simulink model "mdl_GPSreceiveBin1_monitor_v2"  (R2020b)
settings: Solver=FixedStepDiscrete  StartTime=0.0  StopTime=5  FixedStep=0.01  RelTol=1e-3  EnableMultiTasking=on
libraries: simulink x4, raspberrypiCommlib x1
settings Model: ModifiedByFormat=The MathWorks Inc.  SimulationMode=external  EnablePacing=on  Creator=The MathWorks, Inc.  LastModifiedBy=The MathWorks Inc.
settings SolverCC: PositivePriorityOrder=on
settings DataIOCC: SaveFormat=Array  SaveOutput=off  DSMLogging=off  ReturnWorkspaceOutputs=off
settings OptimizationCC: LifeSpan=1  MaxStackSize=64
settings DebuggingCC: UnderspecifiedInitializationDetection=Classic  MergeDetectMultiDrivingBlocksExec=none  SolverPrmCheckMsg=warning  AllowSymbolicDim=off  SFUnexpectedBacktrackingDiag=warning  SFNoUnconditionalDefaultTransitionDiag=warning  SFExecutionAtInitializationDiag=none  ArithmeticOperatorsInVariantConditions=warning
settings HardwareCC: ProdBitPerPointer=32  ProdBitPerSizeT=32  ProdBitPerPtrDiffT=32  ProdLargestAtomicInteger=Long  ProdLargestAtomicFloat=Double  ProdWordSize=32  ProdHWDeviceType=ARM Compatible->ARM Cortex
settings ModelReferenceCC: PropagateSignalLabelsOutOfModel=off
settings SFSimCC: SimUseLocalCustomCode=off  MATLABDynamicMemAlloc=off  CustomCodeUndefinedFunction=UseInterfaceOnly
settings RTWCC: Description=Embedded Coder  SystemTargetFile=ert.tlc  HardwareBoard=Raspberry Pi  TemplateMakefile=ert_default_tmf  RTWVerbose=off  RTWUseLocalCustomCode=off  Toolchain=GNU GCC Raspberry Pi
settings CodeAppCC: MangleLength=10  StateflowObjectComments=on
settings ERTTargetCC: MultiwordLength=2048  ERTCustomFileBanners=off  MatFileLogging=on  SupportContinuousTime=on  RemoveResetFunc=off  SupportVariableSizeSignals=on  ModelStepFunctionPrototypeControlCompliant=off  ExtMode=on  ExtModeTransport=2  ExtModeStaticAlloc=on  ExtModeMexFile=ext_xcp  ExtModeMexArgs='FlexCase04.local' 1 17725  ExtModeIntrfLevel=Level2 - Open  ERTSrcFileBannerTemplate=codertarget_code_template.cgt  ERTHdrFileBannerTemplate=codertarget_code_template.cgt  ERTDataSrcFileTemplate=codertarget_code_template.cgt  ERTDataHdrFileTemplate=codertarget_code_template.cgt  ConvertIfToSwitch=off  SuppressUnreachableDefaultCases=off
settings ConfigComp: CovMetricSettings=dw  CovSaveCumulativeToWorkspaceVar=on  CovSaveSingleToWorkspaceVar=on  CovExternalEMLEnable=off  CovSFcnEnable=off

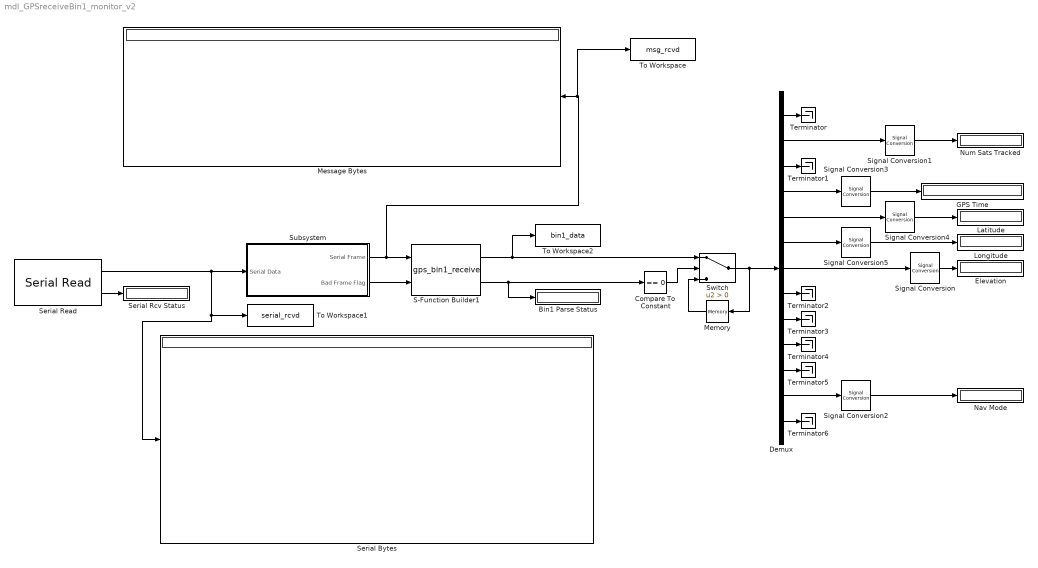
== system mdl_GPSreceiveBin1_monitor_v2 ==
  Bin1 Parse Status : Display
  Compare To Constant : simulink/Logic and Bit Operations/Compare To Constant  relop===  const=0  OutDataTypeStr=uint8
  Demux : Demux  Outputs=13
  Elevation : Display
  GPS Time : Display
      settings: Format=long_e
  Latitude : Display
  Longitude : Display
  Memory : Memory  InheritSampleTime=on  LinearizeAsDelay=on
  Message Bytes : Display
      settings: Format=hex (Stored Integer)
  Nav Mode : Display
  Num Sats Tracked : Display
  S-Function Builder1 : S-Function  FunctionName=gps_bin1_receive  SFunctionModules=gps_bin1_receive_wrapper  SFunctionDeploymentMode=off  EnableBusSupport=off  mask(S-Function Builder){}
      mask help: Simulink:masks:SFunctionBuilder_MD
      mask init:
      | val = [[.9  0.75 0.75 1 1 .9 .9 1]',[1 1 0.75 0.75 .9 .9 1 .9]'];try , sys = get_param(gcb,'SfunBuilderFcnName');if isempty(sys), sys = get_param(gcb,'FunctionName'); end,catch, sys = get_param(gcb,'FunctionName'); end
      settings: CopyFcn=set_param(gcbh,'LinkStatus','none')  OpenFcn=sfunctionwizard(gcbh)
      mask Display:
      | plot(val(:,1),val(:,2))
      | disp(sys)
      | port_label('input',1,'u0')
      | port_label('input',2,'u1')
      | port_label('output',1,'y0')
      | port_label('output',2,'y1')
  Serial Bytes : Display
      settings: Format=hex (Stored Integer)
  Serial Rcv Status : Display
  Serial Read : raspberrypiCommlib/Serial Read  board=Pi 4 Model B  SCIModule_=/dev/serial0  Baudrate_=19200  Parity=None  StopBits_=1  HardwareFlowControl=None  ByteOrder=LittleEndian  DataLength=64  DataType=uint8  OutputStatus=on  SampleTime=-1  blockPlatform=RaspberryPi
      settings: SourceProductBaseCode=RASPPI
  Signal Conversion{,1..5} (6 alike) : SignalConversion  OverrideOpt=off
  Subsystem : Subsystem
  Switch : Switch  Criteria=u2 > Threshold
  Terminator{,1..6} (7 alike) : Terminator
  To Workspace : ToWorkspace  VariableName=msg_rcvd  SampleTime=-1
      settings: Save2DSignal=2-D array (concatenate along first dimension)
  To Workspace1 : ToWorkspace  VariableName=serial_rcvd  SampleTime=-1
      settings: Save2DSignal=2-D array (concatenate along first dimension)
  To Workspace2 : ToWorkspace  VariableName=bin1_data  SampleTime=-1
      settings: Save2DSignal=2-D array (concatenate along first dimension)
  wires:
  Serial Read/2 -> Serial Rcv Status/1
  Demux/2 -> Signal Conversion1/1
  Demux/5 -> Signal Conversion4/1
  Demux/6 -> Signal Conversion5/1
  Demux/7 -> Signal Conversion/1
  Demux/4 -> Signal Conversion3/1
  Demux/1 -> Terminator/1
  Demux/3 -> Terminator1/1
  Demux/8 -> Terminator2/1
  Demux/9 -> Terminator3/1
  Demux/10 -> Terminator4/1
  Demux/11 -> Terminator5/1
  Demux/12 -> Signal Conversion2/1
  Demux/13 -> Terminator6/1
  Signal Conversion/1 -> Elevation/1
  Signal Conversion1/1 -> Num Sats Tracked/1
  Signal Conversion3/1 -> GPS Time/1
  Signal Conversion4/1 -> Latitude/1
  Signal Conversion5/1 -> Longitude/1
  Signal Conversion2/1 -> Nav Mode/1
  Serial Read/1 -> To Workspace1/1, Serial Bytes/1, Subsystem/1(Serial Data)
  Subsystem/2(Bad Frame Flag) -> S-Function Builder1/2
  Subsystem/1(Serial Frame) -> To Workspace/1, Message Bytes/1, S-Function Builder1/1
  S-Function Builder1/2 -> Compare To Constant/1, Bin1 Parse Status/1
  Memory/1 -> Switch/3
  Compare To Constant/1 -> Switch/2
  S-Function Builder1/1 -> Switch/1, To Workspace2/1
  Switch/1 -> Memory/1, Demux/1

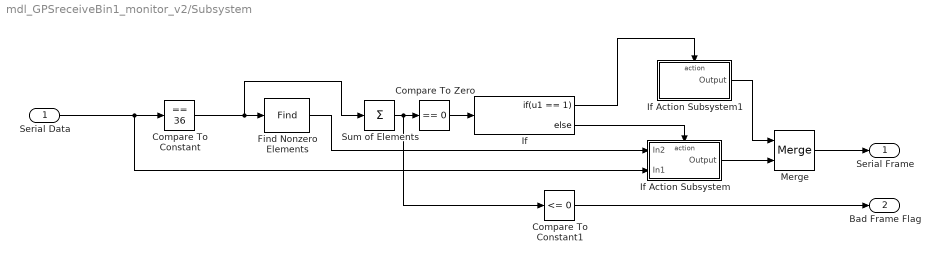
== system mdl_GPSreceiveBin1_monitor_v2/Subsystem ==
  Serial Data : Inport
  Compare To Constant : simulink/Logic and Bit Operations/Compare To Constant  relop===  const=36  OutDataTypeStr=boolean
  Compare To Constant1 : simulink/Logic and Bit Operations/Compare To Constant  relop=<=  const=0  OutDataTypeStr=uint8
  Compare To Zero : simulink/Logic and Bit Operations/Compare To Zero  relop===  OutDataTypeStr=boolean
  Find Nonzero Elements : Find  NumberOfInputDimensions=3
  If : If  IfExpression=u1 == 1
  If Action Subsystem : Subsystem  TreatAsAtomicUnit=on
  If Action Subsystem1 : Subsystem  TreatAsAtomicUnit=on
  Merge : Merge
  Sum of Elements : Sum  Inputs=+
  Serial Frame : Outport
  Bad Frame Flag : Outport  Port=2
  wires:
  Compare To Constant1/1 -> Bad Frame Flag/1
  Find Nonzero Elements/1 -> If Action Subsystem/1(In2)
  Sum of Elements/1 -> Compare To Constant1/1, Compare To Zero/1
  If Action Subsystem1/1(Output) -> Merge/1
  Compare To Constant/1 -> Sum of Elements/1, Find Nonzero Elements/1
  Compare To Zero/1 -> If/1
  If/1 -> If Action Subsystem1/Action
  If/2 -> If Action Subsystem/Action
  If Action Subsystem/1(Output) -> Merge/2
  Serial Data/1 -> If Action Subsystem/2(In1), Compare To Constant/1
  Merge/1 -> Serial Frame/1

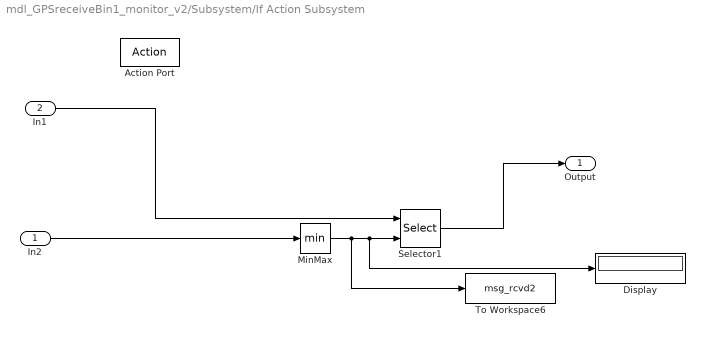
== system mdl_GPSreceiveBin1_monitor_v2/Subsystem/If Action Subsystem ==
  In2 : Inport
  In1 : Inport  Port=2
  Action Port : ActionPort  ActionPortLabel=else
  Display : Display
  MinMax : MinMax
  Selector1 : Selector  InputPortWidth=64  IndexOptions=Starting index (port)  Indices=[1 3]  OutputSizes=64
  To Workspace6 : ToWorkspace  VariableName=msg_rcvd2  SampleTime=-1
      settings: Save2DSignal=2-D array (concatenate along first dimension)
  Output : Outport
  wires:
  Selector1/1 -> Output/1
  In1/1 -> Selector1/1
  MinMax/1 -> Selector1/2, Display/1, To Workspace6/1
  In2/1 -> MinMax/1

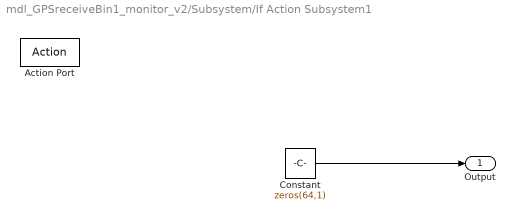
== system mdl_GPSreceiveBin1_monitor_v2/Subsystem/If Action Subsystem1 ==
  Action Port : ActionPort  ActionPortLabel=if(u1 == 1)
  Constant : Constant  Value=zeros(64,1)  OutDataTypeStr=uint8
  Output : Outport
  wires:
  Constant/1 -> Output/1
